simulink model "xor"  (R2015a)
settings: Solver=ode23t  StartTime=0.0  StopTime=1  RelTol=1e-3
libraries: fl_lib x57, nesl_utility x54, elec_lib x5
settings Model: Creator=tomas  LastModifiedBy=tomas

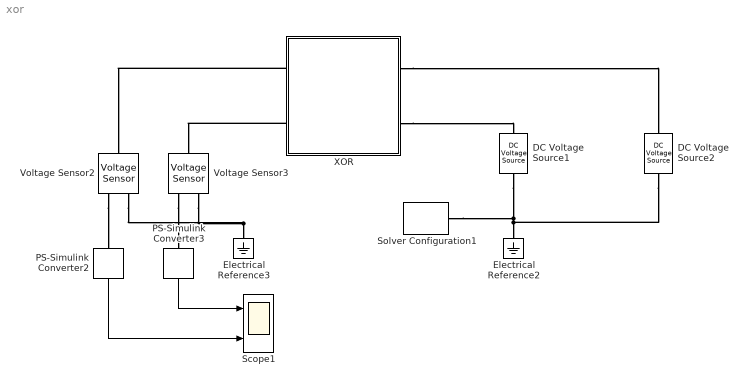
== system xor ==
  DC Voltage Source1 : fl_lib/Electrical/Electrical Sources/DC Voltage Source  v0=1 V
  DC Voltage Source2 : fl_lib/Electrical/Electrical Sources/DC Voltage Source  v0=1 V
  Electrical Reference2 : fl_lib/Electrical/Electrical Elements/Electrical Reference
  Electrical Reference3 : fl_lib/Electrical/Electrical Elements/Electrical Reference
  PS-Simulink Converter2 : nesl_utility/PS-Simulink Converter  PhysicalDomain=network_engine_domain  SubClassName=ps_output  LeftPortType=input  RightPortType=output  PseudoPeriodic=off  Frequencies=[]  Unit=1  AffineConversion=off
  PS-Simulink Converter3 : nesl_utility/PS-Simulink Converter  PhysicalDomain=network_engine_domain  SubClassName=ps_output  LeftPortType=input  RightPortType=output  PseudoPeriodic=off  Frequencies=[]  Unit=1  AffineConversion=off
  Scope1 : Scope  NumInputPorts=2
      settings: YMin=-5~-5  YMax=5~5
  Solver Configuration1 : nesl_utility/Solver Configuration  PhysicalDomain=network_engine_domain  SubClassName=solver  LeftPortType=input  RightPortType=generic  Accelerate=off  Tones=[]  Harmonics=[]  SimulateNoise=off  Profile=off  UseLocalSampling=off  EnableSwitchedLinearOptims=on  FrequencyDomain=off  UseCCode=off  RelTol=0.001  AbsTol=1e-06  MinStep=1e-09  ToWorkspace=off  RevertToSquareIcSolve=off  NumHomotopyIterations=100  DoDC=off  ResidualTolerance=1e-09  UseLocalSolver=off  LocalSolverChoice=NE_BACKWARD_EULER_ADVANCER  LocalSolverSampleTime=0.001  DoFixedCost=off  MaxNonlinIter=3  MaxModeIter=2  LinearAlgebra=Sparse  DelaysMemoryBudget=1024  AutomaticFiltering=on  FilteringTimeConstant=0.001
  Voltage Sensor2 : fl_lib/Electrical/Electrical Sensors/Voltage Sensor
  Voltage Sensor3 : fl_lib/Electrical/Electrical Sensors/Voltage Sensor
  XOR : Subsystem
  wires:
  PS-Simulink Converter3/1 -> Scope1/1
  PS-Simulink Converter2/1 -> Scope1/2
  connections:
  DC Voltage Source1/RConn1 -- Solver Configuration1/RConn1 -- DC Voltage Source2/RConn1 -- Electrical Reference2/LConn1
  Electrical Reference3/LConn1 -- Voltage Sensor3/RConn2 -- Voltage Sensor2/RConn2
  Voltage Sensor2/RConn1 -- PS-Simulink Converter2/LConn1
  XOR/LConn1 -- Voltage Sensor2/LConn1
  XOR/LConn2 -- Voltage Sensor3/LConn1
  Voltage Sensor3/RConn1 -- PS-Simulink Converter3/LConn1
  XOR/RConn2 -- DC Voltage Source1/LConn1
  XOR/RConn1 -- DC Voltage Source2/LConn1

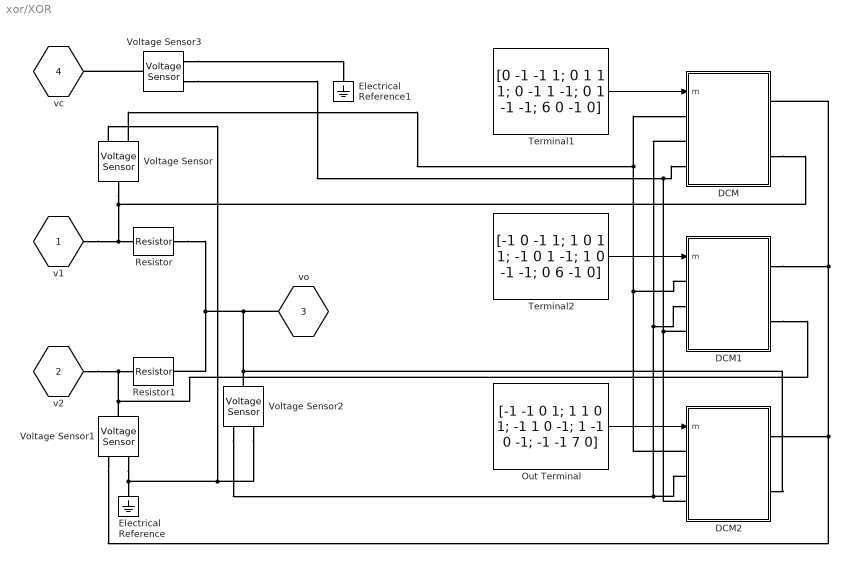
== system xor/XOR ==
  DCM : Subsystem
  DCM1 : Subsystem
  DCM2 : Subsystem
  Electrical Reference : fl_lib/Electrical/Electrical Elements/Electrical Reference
  Electrical Reference1 : fl_lib/Electrical/Electrical Elements/Electrical Reference
  Out Terminal : Constant  Value=[-1 -1 0 1; 1 1 0 1; -1 1 0 -1; 1 -1 0 -1; -1 -1 7 0]  VectorParams1D=off
  Resistor : elec_lib/Passive Devices/Resistor  R=16 kOhm  noise_mode=0  Tdevice=25 C  sample_time=0.001 s  repeatability=1  auto_seed=3002755773  user_seed=0
  Resistor1 : elec_lib/Passive Devices/Resistor  R=16 kOhm  noise_mode=0  Tdevice=25 C  sample_time=0.001 s  repeatability=1  auto_seed=3419901825  user_seed=0
  Terminal1 : Constant  Value=[0 -1 -1 1; 0 1 1 1; 0 -1 1 -1; 0 1 -1 -1; 6 0 -1 0]  VectorParams1D=off
  Terminal2 : Constant  Value=[-1 0 -1 1; 1 0 1 1; -1 0 1 -1; 1 0 -1 -1; 0 6 -1 0]  VectorParams1D=off
  Voltage Sensor{,1..3} (4 alike) : fl_lib/Electrical/Electrical Sensors/Voltage Sensor
  v1 : PMIOPort  Port=1  Side=Left
  v2 : PMIOPort  Port=2  Side=Left
  vo : PMIOPort  Port=3  Side=Right
  vc : PMIOPort  Port=4  Side=Right
  wires:
  Terminal2/1 -> DCM1/1(m)
  Out Terminal/1 -> DCM2/1(m)
  Terminal1/1 -> DCM/1(m)
  connections:
  DCM/RConn2 -- Voltage Sensor/LConn1 -- Resistor/LConn1 -- v1/RConn1
  DCM1/RConn2 -- Voltage Sensor1/LConn1 -- Resistor1/LConn1 -- v2/RConn1
  DCM2/RConn1 -- DCM1/RConn1 -- DCM/RConn1 -- Voltage Sensor1/RConn1
  DCM2/LConn1 -- DCM1/LConn1 -- DCM/LConn1 -- Voltage Sensor/RConn1
  DCM2/RConn2 -- Voltage Sensor2/LConn1 -- Resistor/RConn1 -- Resistor1/RConn1 -- vo/RConn1
  Voltage Sensor2/RConn2 -- Voltage Sensor1/RConn2 -- Electrical Reference/LConn1 -- Voltage Sensor/RConn2
  DCM2/LConn2 -- DCM/LConn2 -- DCM1/LConn2 -- Voltage Sensor2/RConn1
  Voltage Sensor3/LConn1 -- vc/RConn1
  DCM1/LConn3 -- DCM/LConn3 -- Voltage Sensor3/RConn1 -- DCM2/LConn3
  Voltage Sensor3/RConn2 -- Electrical Reference1/LConn1

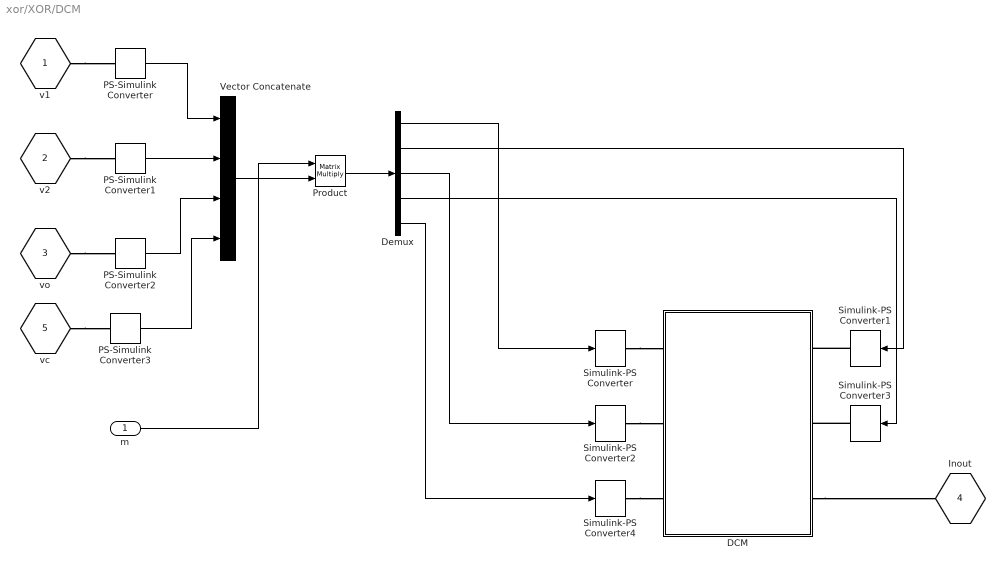
== system xor/XOR/DCM ==
  m : Inport
  DCM : Subsystem
  Demux : Demux  Outputs=5
  PS-Simulink Converter{,1..3} (4 alike) : nesl_utility/PS-Simulink Converter  PhysicalDomain=network_engine_domain  SubClassName=ps_output  LeftPortType=input  RightPortType=output  PseudoPeriodic=off  Frequencies=[]  Unit=V  AffineConversion=off
  Product : Product  Multiplication=Matrix(*)
  Simulink-PS Converter{,1..4} (5 alike) : nesl_utility/Simulink-PS Converter  PhysicalDomain=network_engine_domain  SubClassName=ps_input  LeftPortType=input  RightPortType=output  PseudoPeriodic=off  Frequencies=[]  NoiseDistribution=none  NoiseParameters=[]  Unit=V  AffineConversion=off  InputFiltering=off  SimscapeFilterOrder=1  InputFilterTimeConstant=0.001  UdotUserProvided=1
  Vector Concatenate : Concatenate  NumInputs=4
  "v1 " : PMIOPort  Port=1  Side=Left
  v2 : PMIOPort  Port=2  Side=Right
  vo : PMIOPort  Port=3  Side=Left
  Inout : PMIOPort  Port=4  Side=Right
  vc : PMIOPort  Port=5  Side=Left
  wires:
  Demux/5 -> Simulink-PS Converter4/1
  PS-Simulink Converter3/1 -> Vector Concatenate/4
  Demux/3 -> Simulink-PS Converter2/1
  PS-Simulink Converter/1 -> Vector Concatenate/1
  PS-Simulink Converter2/1 -> Vector Concatenate/3
  PS-Simulink Converter1/1 -> Vector Concatenate/2
  Demux/1 -> Simulink-PS Converter/1
  Demux/4 -> Simulink-PS Converter3/1
  m/1 -> Product/1
  Vector Concatenate/1 -> Product/2
  Product/1 -> Demux/1
  Demux/2 -> Simulink-PS Converter1/1
  connections:
  Simulink-PS Converter2/RConn1 -- DCM/LConn2
  DCM/RConn3 -- Inout/RConn1
  Simulink-PS Converter3/RConn1 -- DCM/RConn2
  vo/RConn1 -- PS-Simulink Converter2/LConn1
  Simulink-PS Converter4/RConn1 -- DCM/LConn3
  Simulink-PS Converter/RConn1 -- DCM/LConn1
  "v1 "/RConn1 -- PS-Simulink Converter/LConn1
  v2/RConn1 -- PS-Simulink Converter1/LConn1
  Simulink-PS Converter1/RConn1 -- DCM/RConn1
  vc/RConn1 -- PS-Simulink Converter3/LConn1

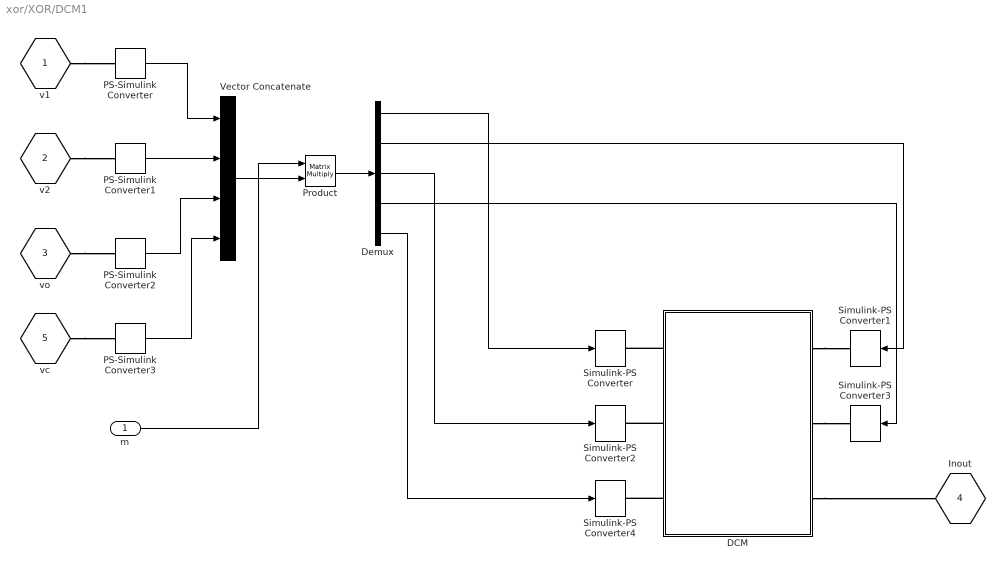
== system xor/XOR/DCM1 ==
  m : Inport
  DCM : Subsystem
  Demux : Demux  Outputs=5
  PS-Simulink Converter{,1..3} (4 alike) : nesl_utility/PS-Simulink Converter  PhysicalDomain=network_engine_domain  SubClassName=ps_output  LeftPortType=input  RightPortType=output  PseudoPeriodic=off  Frequencies=[]  Unit=V  AffineConversion=off
  Product : Product  Multiplication=Matrix(*)
  Simulink-PS Converter{,1..4} (5 alike) : nesl_utility/Simulink-PS Converter  PhysicalDomain=network_engine_domain  SubClassName=ps_input  LeftPortType=input  RightPortType=output  PseudoPeriodic=off  Frequencies=[]  NoiseDistribution=none  NoiseParameters=[]  Unit=V  AffineConversion=off  InputFiltering=off  SimscapeFilterOrder=1  InputFilterTimeConstant=0.001  UdotUserProvided=1
  Vector Concatenate : Concatenate  NumInputs=4
  "v1 " : PMIOPort  Port=1  Side=Left
  v2 : PMIOPort  Port=2  Side=Right
  vo : PMIOPort  Port=3  Side=Left
  Inout : PMIOPort  Port=4  Side=Right
  vc : PMIOPort  Port=5  Side=Left
  wires:
  Demux/5 -> Simulink-PS Converter4/1
  Demux/3 -> Simulink-PS Converter2/1
  PS-Simulink Converter/1 -> Vector Concatenate/1
  PS-Simulink Converter2/1 -> Vector Concatenate/3
  Demux/2 -> Simulink-PS Converter1/1
  PS-Simulink Converter1/1 -> Vector Concatenate/2
  Demux/1 -> Simulink-PS Converter/1
  Demux/4 -> Simulink-PS Converter3/1
  m/1 -> Product/1
  Vector Concatenate/1 -> Product/2
  Product/1 -> Demux/1
  PS-Simulink Converter3/1 -> Vector Concatenate/4
  connections:
  DCM/LConn2 -- Simulink-PS Converter2/RConn1
  vo/RConn1 -- PS-Simulink Converter2/LConn1
  DCM/LConn3 -- Simulink-PS Converter4/RConn1
  DCM/LConn1 -- Simulink-PS Converter/RConn1
  "v1 "/RConn1 -- PS-Simulink Converter/LConn1
  v2/RConn1 -- PS-Simulink Converter1/LConn1
  vc/RConn1 -- PS-Simulink Converter3/LConn1
  DCM/RConn1 -- Simulink-PS Converter1/RConn1
  DCM/RConn2 -- Simulink-PS Converter3/RConn1
  DCM/RConn3 -- Inout/RConn1

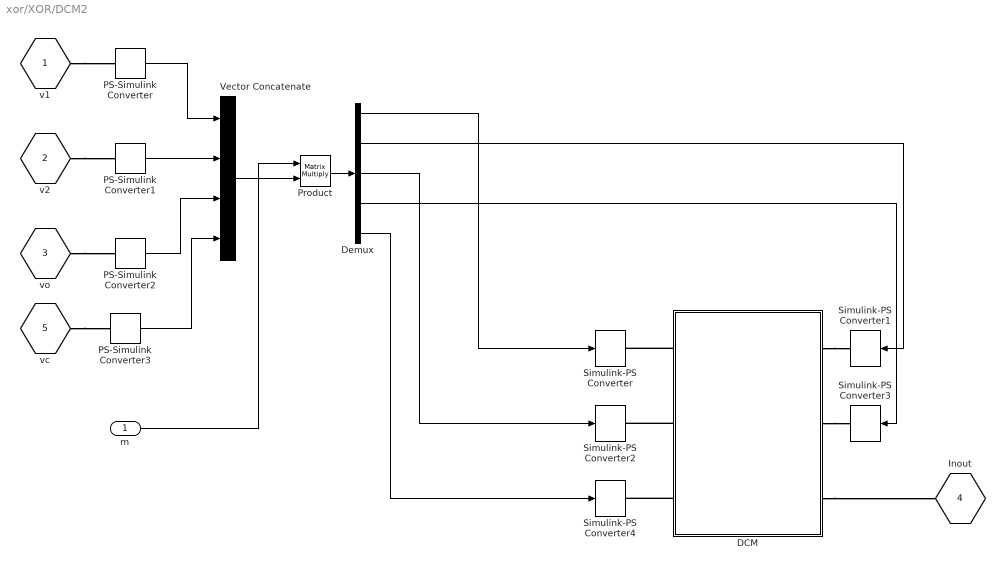
== system xor/XOR/DCM2 ==
  m : Inport
  DCM : Subsystem
  Demux : Demux  Outputs=5
  PS-Simulink Converter{,1..3} (4 alike) : nesl_utility/PS-Simulink Converter  PhysicalDomain=network_engine_domain  SubClassName=ps_output  LeftPortType=input  RightPortType=output  PseudoPeriodic=off  Frequencies=[]  Unit=V  AffineConversion=off
  Product : Product  Multiplication=Matrix(*)
  Simulink-PS Converter{,1..4} (5 alike) : nesl_utility/Simulink-PS Converter  PhysicalDomain=network_engine_domain  SubClassName=ps_input  LeftPortType=input  RightPortType=output  PseudoPeriodic=off  Frequencies=[]  NoiseDistribution=none  NoiseParameters=[]  Unit=V  AffineConversion=off  InputFiltering=off  SimscapeFilterOrder=1  InputFilterTimeConstant=0.001  UdotUserProvided=1
  Vector Concatenate : Concatenate  NumInputs=4
  "v1 " : PMIOPort  Port=1  Side=Left
  v2 : PMIOPort  Port=2  Side=Right
  vo : PMIOPort  Port=3  Side=Left
  Inout : PMIOPort  Port=4  Side=Right
  vc : PMIOPort  Port=5  Side=Left
  wires:
  Demux/5 -> Simulink-PS Converter4/1
  Demux/3 -> Simulink-PS Converter2/1
  PS-Simulink Converter/1 -> Vector Concatenate/1
  PS-Simulink Converter2/1 -> Vector Concatenate/3
  Demux/2 -> Simulink-PS Converter1/1
  PS-Simulink Converter1/1 -> Vector Concatenate/2
  Demux/1 -> Simulink-PS Converter/1
  Demux/4 -> Simulink-PS Converter3/1
  m/1 -> Product/1
  Vector Concatenate/1 -> Product/2
  Product/1 -> Demux/1
  PS-Simulink Converter3/1 -> Vector Concatenate/4
  connections:
  DCM/LConn2 -- Simulink-PS Converter2/RConn1
  vo/RConn1 -- PS-Simulink Converter2/LConn1
  DCM/LConn3 -- Simulink-PS Converter4/RConn1
  DCM/LConn1 -- Simulink-PS Converter/RConn1
  "v1 "/RConn1 -- PS-Simulink Converter/LConn1
  v2/RConn1 -- PS-Simulink Converter1/LConn1
  vc/RConn1 -- PS-Simulink Converter3/LConn1
  DCM/RConn1 -- Simulink-PS Converter1/RConn1
  DCM/RConn2 -- Simulink-PS Converter3/RConn1
  DCM/RConn3 -- Inout/RConn1

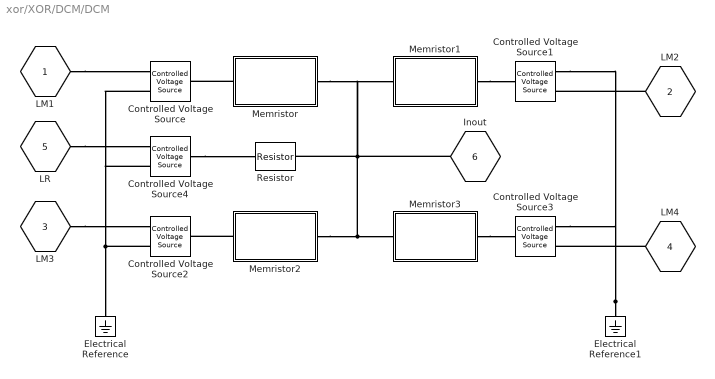
== system xor/XOR/DCM/DCM ==
  Controlled Voltage Source{,1..4} (5 alike) : fl_lib/Electrical/Electrical Sources/Controlled Voltage Source
  Electrical Reference : fl_lib/Electrical/Electrical Elements/Electrical Reference
  Electrical Reference1 : fl_lib/Electrical/Electrical Elements/Electrical Reference
  Memristor : Subsystem  Tag=Memristor
  Memristor1 : Subsystem  Tag=Memristor
  Memristor2 : Subsystem  Tag=Memristor
  Memristor3 : Subsystem  Tag=Memristor
  Resistor : elec_lib/Passive Devices/Resistor  R=16 kOhm  noise_mode=0  Tdevice=25 C  sample_time=0.001 s  repeatability=1  auto_seed=2451064179  user_seed=0
  LM1 : PMIOPort  Port=1  Side=Left
  LM2 : PMIOPort  Port=2  Side=Right
  LM3 : PMIOPort  Port=3  Side=Left
  LM4 : PMIOPort  Port=4  Side=Right
  LR : PMIOPort  Port=5  Side=Left
  Inout : PMIOPort  Port=6  Side=Right
  connections:
  LM2/RConn1 -- Controlled Voltage Source1/RConn1
  Controlled Voltage Source2/RConn2 -- Electrical Reference/LConn1 -- Controlled Voltage Source/RConn2 -- Controlled Voltage Source4/RConn2
  Controlled Voltage Source4/LConn1 -- Resistor/LConn1
  Memristor2/RConn1 -- Memristor1/LConn1 -- Memristor/LConn1 -- Resistor/RConn1 -- Inout/RConn1 -- Memristor3/RConn1
  Electrical Reference1/LConn1 -- Controlled Voltage Source1/RConn2 -- Controlled Voltage Source3/RConn2
  LM1/RConn1 -- Controlled Voltage Source/RConn1
  LM4/RConn1 -- Controlled Voltage Source3/RConn1
  LR/RConn1 -- Controlled Voltage Source4/RConn1
  LM3/RConn1 -- Controlled Voltage Source2/RConn1
  Memristor2/LConn1 -- Controlled Voltage Source2/LConn1
  Memristor3/LConn1 -- Controlled Voltage Source3/LConn1
  Memristor1/RConn1 -- Controlled Voltage Source1/LConn1
  Memristor/RConn1 -- Controlled Voltage Source/LConn1

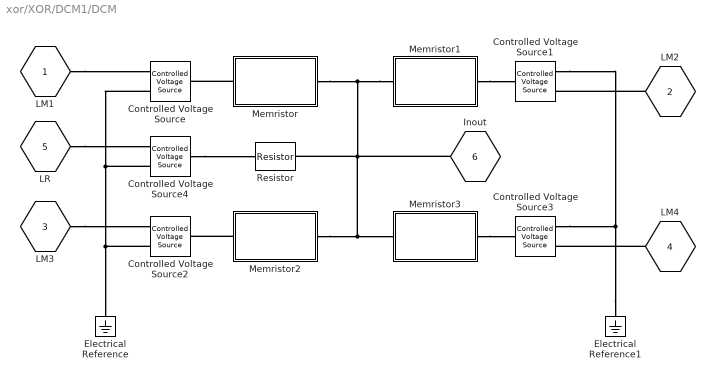
== system xor/XOR/DCM1/DCM ==
  Controlled Voltage Source{,1..4} (5 alike) : fl_lib/Electrical/Electrical Sources/Controlled Voltage Source
  Electrical Reference : fl_lib/Electrical/Electrical Elements/Electrical Reference
  Electrical Reference1 : fl_lib/Electrical/Electrical Elements/Electrical Reference
  Memristor : Subsystem  Tag=Memristor
  Memristor1 : Subsystem  Tag=Memristor
  Memristor2 : Subsystem  Tag=Memristor
  Memristor3 : Subsystem  Tag=Memristor
  Resistor : elec_lib/Passive Devices/Resistor  R=16 kOhm  noise_mode=0  Tdevice=25 C  sample_time=0.001 s  repeatability=1  auto_seed=1880221209  user_seed=0
  LM1 : PMIOPort  Port=1  Side=Left
  LM2 : PMIOPort  Port=2  Side=Right
  LM3 : PMIOPort  Port=3  Side=Left
  LM4 : PMIOPort  Port=4  Side=Right
  LR : PMIOPort  Port=5  Side=Left
  Inout : PMIOPort  Port=6  Side=Right
  connections:
  LM2/RConn1 -- Controlled Voltage Source1/RConn1
  Controlled Voltage Source2/RConn2 -- Electrical Reference/LConn1 -- Controlled Voltage Source/RConn2 -- Controlled Voltage Source4/RConn2
  Controlled Voltage Source4/LConn1 -- Resistor/LConn1
  Memristor1/LConn1 -- Memristor/LConn1 -- Resistor/RConn1 -- Inout/RConn1 -- Memristor2/RConn1 -- Memristor3/RConn1
  Electrical Reference1/LConn1 -- Controlled Voltage Source1/RConn2 -- Controlled Voltage Source3/RConn2
  LM1/RConn1 -- Controlled Voltage Source/RConn1
  LM4/RConn1 -- Controlled Voltage Source3/RConn1
  LR/RConn1 -- Controlled Voltage Source4/RConn1
  LM3/RConn1 -- Controlled Voltage Source2/RConn1
  Memristor2/LConn1 -- Controlled Voltage Source2/LConn1
  Memristor3/LConn1 -- Controlled Voltage Source3/LConn1
  Memristor1/RConn1 -- Controlled Voltage Source1/LConn1
  Memristor/RConn1 -- Controlled Voltage Source/LConn1

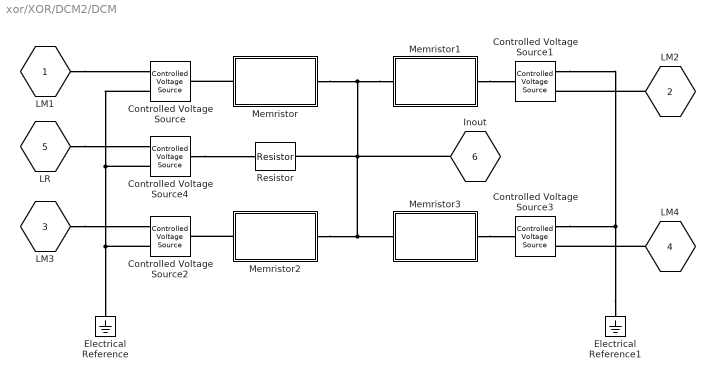
== system xor/XOR/DCM2/DCM ==
  Controlled Voltage Source{,1..4} (5 alike) : fl_lib/Electrical/Electrical Sources/Controlled Voltage Source
  Electrical Reference : fl_lib/Electrical/Electrical Elements/Electrical Reference
  Electrical Reference1 : fl_lib/Electrical/Electrical Elements/Electrical Reference
  Memristor : Subsystem  Tag=Memristor
  Memristor1 : Subsystem  Tag=Memristor
  Memristor2 : Subsystem  Tag=Memristor
  Memristor3 : Subsystem  Tag=Memristor
  Resistor : elec_lib/Passive Devices/Resistor  R=16 kOhm  noise_mode=0  Tdevice=25 C  sample_time=0.001 s  repeatability=1  auto_seed=1203579070  user_seed=0
  LM1 : PMIOPort  Port=1  Side=Left
  LM2 : PMIOPort  Port=2  Side=Right
  LM3 : PMIOPort  Port=3  Side=Left
  LM4 : PMIOPort  Port=4  Side=Right
  LR : PMIOPort  Port=5  Side=Left
  Inout : PMIOPort  Port=6  Side=Right
  connections:
  LM2/RConn1 -- Controlled Voltage Source1/RConn1
  Controlled Voltage Source2/RConn2 -- Electrical Reference/LConn1 -- Controlled Voltage Source/RConn2 -- Controlled Voltage Source4/RConn2
  Controlled Voltage Source4/LConn1 -- Resistor/LConn1
  Memristor1/LConn1 -- Memristor/LConn1 -- Resistor/RConn1 -- Inout/RConn1 -- Memristor2/RConn1 -- Memristor3/RConn1
  Electrical Reference1/LConn1 -- Controlled Voltage Source1/RConn2 -- Controlled Voltage Source3/RConn2
  LM1/RConn1 -- Controlled Voltage Source/RConn1
  LM4/RConn1 -- Controlled Voltage Source3/RConn1
  LR/RConn1 -- Controlled Voltage Source4/RConn1
  LM3/RConn1 -- Controlled Voltage Source2/RConn1
  Memristor2/LConn1 -- Controlled Voltage Source2/LConn1
  Memristor3/LConn1 -- Controlled Voltage Source3/LConn1
  Memristor1/RConn1 -- Controlled Voltage Source1/LConn1
  Memristor/RConn1 -- Controlled Voltage Source/LConn1

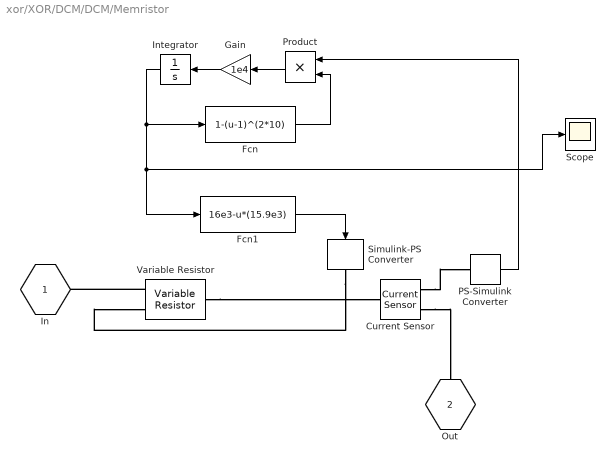
== system xor/XOR/DCM/DCM/Memristor ==
  Current Sensor : fl_lib/Electrical/Electrical Sensors/Current Sensor
  Fcn : Fcn  Expr=1-(u-1)^(2*10)
  Fcn1 : Fcn  Expr=16e3-u*(15.9e3)
  Gain : Gain  Gain=1e4
  Integrator : Integrator  InitialCondition=rand()
  PS-Simulink Converter : nesl_utility/PS-Simulink Converter  PhysicalDomain=network_engine_domain  SubClassName=ps_output  LeftPortType=input  RightPortType=output  PseudoPeriodic=off  Frequencies=[]  Unit=1  AffineConversion=off
  Product : Product
  Scope : Scope
  Simulink-PS Converter : nesl_utility/Simulink-PS Converter  PhysicalDomain=network_engine_domain  SubClassName=ps_input  LeftPortType=input  RightPortType=output  PseudoPeriodic=off  Frequencies=[]  NoiseDistribution=none  NoiseParameters=[]  Unit=1  AffineConversion=off  InputFiltering=off  SimscapeFilterOrder=1  InputFilterTimeConstant=0.001  UdotUserProvided=1
  Variable Resistor : fl_lib/Electrical/Electrical Elements/Variable Resistor  Rmin=100 Ohm  i_specify=off  i_priority=High  i=0 A  v_specify=off  v_priority=High  v=0 V
  In : PMIOPort  Port=1  Side=Left
  Out : PMIOPort  Port=2  Side=Right
  wires:
  Gain/1 -> Integrator/1
  Product/1 -> Gain/1
  Integrator/1 -> Scope/1, Fcn1/1, Fcn/1
  Fcn/1 -> Product/2
  Fcn1/1 -> Simulink-PS Converter/1
  PS-Simulink Converter/1 -> Product/1
  connections:
  Current Sensor/RConn1 -- PS-Simulink Converter/LConn1
  Simulink-PS Converter/RConn1 -- Variable Resistor/LConn1
  Current Sensor/RConn2 -- Out/RConn1
  Variable Resistor/RConn1 -- Current Sensor/LConn1
  Variable Resistor/LConn2 -- In/RConn1

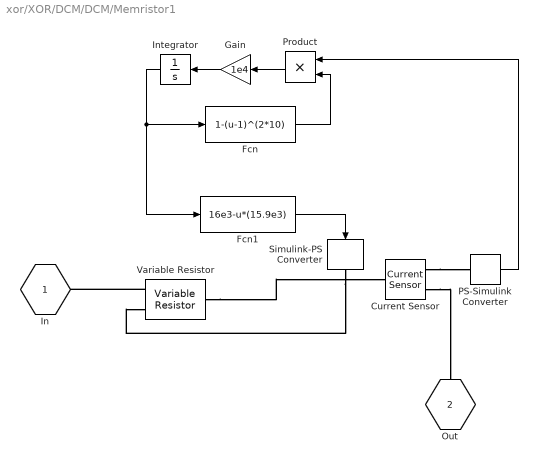
== system xor/XOR/DCM/DCM/Memristor1 ==
  Current Sensor : fl_lib/Electrical/Electrical Sensors/Current Sensor
  Fcn : Fcn  Expr=1-(u-1)^(2*10)
  Fcn1 : Fcn  Expr=16e3-u*(15.9e3)
  Gain : Gain  Gain=1e4
  Integrator : Integrator  InitialCondition=rand()
  PS-Simulink Converter : nesl_utility/PS-Simulink Converter  PhysicalDomain=network_engine_domain  SubClassName=ps_output  LeftPortType=input  RightPortType=output  PseudoPeriodic=off  Frequencies=[]  Unit=1  AffineConversion=off
  Product : Product
  Simulink-PS Converter : nesl_utility/Simulink-PS Converter  PhysicalDomain=network_engine_domain  SubClassName=ps_input  LeftPortType=input  RightPortType=output  PseudoPeriodic=off  Frequencies=[]  NoiseDistribution=none  NoiseParameters=[]  Unit=1  AffineConversion=off  InputFiltering=off  SimscapeFilterOrder=1  InputFilterTimeConstant=0.001  UdotUserProvided=1
  Variable Resistor : fl_lib/Electrical/Electrical Elements/Variable Resistor  Rmin=100 Ohm  i_specify=off  i_priority=High  i=0 A  v_specify=off  v_priority=High  v=0 V
  In : PMIOPort  Port=1  Side=Left
  Out : PMIOPort  Port=2  Side=Right
  wires:
  Gain/1 -> Integrator/1
  Product/1 -> Gain/1
  Integrator/1 -> Fcn1/1, Fcn/1
  Fcn/1 -> Product/2
  Fcn1/1 -> Simulink-PS Converter/1
  PS-Simulink Converter/1 -> Product/1
  connections:
  Variable Resistor/LConn2 -- In/RConn1
  Current Sensor/RConn1 -- PS-Simulink Converter/LConn1
  Current Sensor/RConn2 -- Out/RConn1
  Simulink-PS Converter/RConn1 -- Variable Resistor/LConn1
  Variable Resistor/RConn1 -- Current Sensor/LConn1

== system xor/XOR/DCM/DCM/Memristor2 ==
  Current Sensor : fl_lib/Electrical/Electrical Sensors/Current Sensor
  Fcn : Fcn  Expr=1-(u-1)^(2*10)
  Fcn1 : Fcn  Expr=16e3-u*(15.9e3)
  Gain : Gain  Gain=1e4
  Integrator : Integrator  InitialCondition=rand()
  PS-Simulink Converter : nesl_utility/PS-Simulink Converter  PhysicalDomain=network_engine_domain  SubClassName=ps_output  LeftPortType=input  RightPortType=output  PseudoPeriodic=off  Frequencies=[]  Unit=1  AffineConversion=off
  Product : Product
  Simulink-PS Converter : nesl_utility/Simulink-PS Converter  PhysicalDomain=network_engine_domain  SubClassName=ps_input  LeftPortType=input  RightPortType=output  PseudoPeriodic=off  Frequencies=[]  NoiseDistribution=none  NoiseParameters=[]  Unit=1  AffineConversion=off  InputFiltering=off  SimscapeFilterOrder=1  InputFilterTimeConstant=0.001  UdotUserProvided=1
  Variable Resistor : fl_lib/Electrical/Electrical Elements/Variable Resistor  Rmin=100 Ohm  i_specify=off  i_priority=High  i=0 A  v_specify=off  v_priority=High  v=0 V
  In : PMIOPort  Port=1  Side=Left
  Out : PMIOPort  Port=2  Side=Right
  wires:
  Gain/1 -> Integrator/1
  Product/1 -> Gain/1
  Integrator/1 -> Fcn1/1, Fcn/1
  Fcn/1 -> Product/2
  Fcn1/1 -> Simulink-PS Converter/1
  PS-Simulink Converter/1 -> Product/1
  connections:
  Variable Resistor/LConn2 -- In/RConn1
  Current Sensor/RConn1 -- PS-Simulink Converter/LConn1
  Current Sensor/RConn2 -- Out/RConn1
  Variable Resistor/RConn1 -- Current Sensor/LConn1
  Simulink-PS Converter/RConn1 -- Variable Resistor/LConn1

== system xor/XOR/DCM/DCM/Memristor3 ==
  Current Sensor : fl_lib/Electrical/Electrical Sensors/Current Sensor
  Fcn : Fcn  Expr=1-(u-1)^(2*10)
  Fcn1 : Fcn  Expr=16e3-u*(15.9e3)
  Gain : Gain  Gain=1e4
  Integrator : Integrator  InitialCondition=rand()
  PS-Simulink Converter : nesl_utility/PS-Simulink Converter  PhysicalDomain=network_engine_domain  SubClassName=ps_output  LeftPortType=input  RightPortType=output  PseudoPeriodic=off  Frequencies=[]  Unit=1  AffineConversion=off
  Product : Product
  Simulink-PS Converter : nesl_utility/Simulink-PS Converter  PhysicalDomain=network_engine_domain  SubClassName=ps_input  LeftPortType=input  RightPortType=output  PseudoPeriodic=off  Frequencies=[]  NoiseDistribution=none  NoiseParameters=[]  Unit=1  AffineConversion=off  InputFiltering=off  SimscapeFilterOrder=1  InputFilterTimeConstant=0.001  UdotUserProvided=1
  Variable Resistor : fl_lib/Electrical/Electrical Elements/Variable Resistor  Rmin=100 Ohm  i_specify=off  i_priority=High  i=0 A  v_specify=off  v_priority=High  v=0 V
  In : PMIOPort  Port=1  Side=Left
  Out : PMIOPort  Port=2  Side=Right
  wires:
  Gain/1 -> Integrator/1
  Product/1 -> Gain/1
  Integrator/1 -> Fcn1/1, Fcn/1
  Fcn/1 -> Product/2
  Fcn1/1 -> Simulink-PS Converter/1
  PS-Simulink Converter/1 -> Product/1
  connections:
  Current Sensor/RConn1 -- PS-Simulink Converter/LConn1
  Current Sensor/RConn2 -- Out/RConn1
  Variable Resistor/LConn2 -- In/RConn1
  Simulink-PS Converter/RConn1 -- Variable Resistor/LConn1
  Variable Resistor/RConn1 -- Current Sensor/LConn1

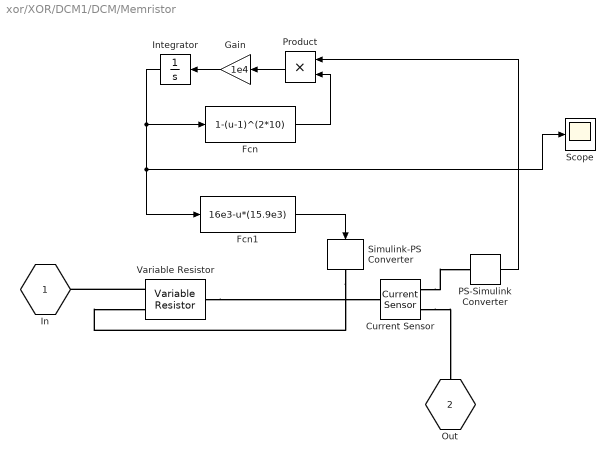
== system xor/XOR/DCM1/DCM/Memristor ==
  Current Sensor : fl_lib/Electrical/Electrical Sensors/Current Sensor
  Fcn : Fcn  Expr=1-(u-1)^(2*10)
  Fcn1 : Fcn  Expr=16e3-u*(15.9e3)
  Gain : Gain  Gain=1e4
  Integrator : Integrator  InitialCondition=rand()
  PS-Simulink Converter : nesl_utility/PS-Simulink Converter  PhysicalDomain=network_engine_domain  SubClassName=ps_output  LeftPortType=input  RightPortType=output  PseudoPeriodic=off  Frequencies=[]  Unit=1  AffineConversion=off
  Product : Product
  Scope : Scope
  Simulink-PS Converter : nesl_utility/Simulink-PS Converter  PhysicalDomain=network_engine_domain  SubClassName=ps_input  LeftPortType=input  RightPortType=output  PseudoPeriodic=off  Frequencies=[]  NoiseDistribution=none  NoiseParameters=[]  Unit=1  AffineConversion=off  InputFiltering=off  SimscapeFilterOrder=1  InputFilterTimeConstant=0.001  UdotUserProvided=1
  Variable Resistor : fl_lib/Electrical/Electrical Elements/Variable Resistor  Rmin=100 Ohm  i_specify=off  i_priority=High  i=0 A  v_specify=off  v_priority=High  v=0 V
  In : PMIOPort  Port=1  Side=Left
  Out : PMIOPort  Port=2  Side=Right
  wires:
  Gain/1 -> Integrator/1
  Product/1 -> Gain/1
  Integrator/1 -> Scope/1, Fcn1/1, Fcn/1
  Fcn/1 -> Product/2
  Fcn1/1 -> Simulink-PS Converter/1
  PS-Simulink Converter/1 -> Product/1
  connections:
  Current Sensor/RConn1 -- PS-Simulink Converter/LConn1
  Simulink-PS Converter/RConn1 -- Variable Resistor/LConn1
  Current Sensor/RConn2 -- Out/RConn1
  Variable Resistor/RConn1 -- Current Sensor/LConn1
  Variable Resistor/LConn2 -- In/RConn1

== system xor/XOR/DCM1/DCM/Memristor1 ==
  Current Sensor : fl_lib/Electrical/Electrical Sensors/Current Sensor
  Fcn : Fcn  Expr=1-(u-1)^(2*10)
  Fcn1 : Fcn  Expr=16e3-u*(15.9e3)
  Gain : Gain  Gain=1e4
  Integrator : Integrator  InitialCondition=rand()
  PS-Simulink Converter : nesl_utility/PS-Simulink Converter  PhysicalDomain=network_engine_domain  SubClassName=ps_output  LeftPortType=input  RightPortType=output  PseudoPeriodic=off  Frequencies=[]  Unit=1  AffineConversion=off
  Product : Product
  Simulink-PS Converter : nesl_utility/Simulink-PS Converter  PhysicalDomain=network_engine_domain  SubClassName=ps_input  LeftPortType=input  RightPortType=output  PseudoPeriodic=off  Frequencies=[]  NoiseDistribution=none  NoiseParameters=[]  Unit=1  AffineConversion=off  InputFiltering=off  SimscapeFilterOrder=1  InputFilterTimeConstant=0.001  UdotUserProvided=1
  Variable Resistor : fl_lib/Electrical/Electrical Elements/Variable Resistor  Rmin=100 Ohm  i_specify=off  i_priority=High  i=0 A  v_specify=off  v_priority=High  v=0 V
  In : PMIOPort  Port=1  Side=Left
  Out : PMIOPort  Port=2  Side=Right
  wires:
  Gain/1 -> Integrator/1
  Product/1 -> Gain/1
  Integrator/1 -> Fcn1/1, Fcn/1
  Fcn/1 -> Product/2
  Fcn1/1 -> Simulink-PS Converter/1
  PS-Simulink Converter/1 -> Product/1
  connections:
  Variable Resistor/LConn2 -- In/RConn1
  Current Sensor/RConn1 -- PS-Simulink Converter/LConn1
  Current Sensor/RConn2 -- Out/RConn1
  Simulink-PS Converter/RConn1 -- Variable Resistor/LConn1
  Variable Resistor/RConn1 -- Current Sensor/LConn1

== system xor/XOR/DCM1/DCM/Memristor2 ==
  Current Sensor : fl_lib/Electrical/Electrical Sensors/Current Sensor
  Fcn : Fcn  Expr=1-(u-1)^(2*10)
  Fcn1 : Fcn  Expr=16e3-u*(15.9e3)
  Gain : Gain  Gain=1e4
  Integrator : Integrator  InitialCondition=rand()
  PS-Simulink Converter : nesl_utility/PS-Simulink Converter  PhysicalDomain=network_engine_domain  SubClassName=ps_output  LeftPortType=input  RightPortType=output  PseudoPeriodic=off  Frequencies=[]  Unit=1  AffineConversion=off
  Product : Product
  Simulink-PS Converter : nesl_utility/Simulink-PS Converter  PhysicalDomain=network_engine_domain  SubClassName=ps_input  LeftPortType=input  RightPortType=output  PseudoPeriodic=off  Frequencies=[]  NoiseDistribution=none  NoiseParameters=[]  Unit=1  AffineConversion=off  InputFiltering=off  SimscapeFilterOrder=1  InputFilterTimeConstant=0.001  UdotUserProvided=1
  Variable Resistor : fl_lib/Electrical/Electrical Elements/Variable Resistor  Rmin=100 Ohm  i_specify=off  i_priority=High  i=0 A  v_specify=off  v_priority=High  v=0 V
  In : PMIOPort  Port=1  Side=Left
  Out : PMIOPort  Port=2  Side=Right
  wires:
  Gain/1 -> Integrator/1
  Product/1 -> Gain/1
  Integrator/1 -> Fcn1/1, Fcn/1
  Fcn/1 -> Product/2
  Fcn1/1 -> Simulink-PS Converter/1
  PS-Simulink Converter/1 -> Product/1
  connections:
  Variable Resistor/LConn2 -- In/RConn1
  Current Sensor/RConn1 -- PS-Simulink Converter/LConn1
  Current Sensor/RConn2 -- Out/RConn1
  Variable Resistor/RConn1 -- Current Sensor/LConn1
  Simulink-PS Converter/RConn1 -- Variable Resistor/LConn1

== system xor/XOR/DCM1/DCM/Memristor3 ==
  Current Sensor : fl_lib/Electrical/Electrical Sensors/Current Sensor
  Fcn : Fcn  Expr=1-(u-1)^(2*10)
  Fcn1 : Fcn  Expr=16e3-u*(15.9e3)
  Gain : Gain  Gain=1e4
  Integrator : Integrator  InitialCondition=rand()
  PS-Simulink Converter : nesl_utility/PS-Simulink Converter  PhysicalDomain=network_engine_domain  SubClassName=ps_output  LeftPortType=input  RightPortType=output  PseudoPeriodic=off  Frequencies=[]  Unit=1  AffineConversion=off
  Product : Product
  Simulink-PS Converter : nesl_utility/Simulink-PS Converter  PhysicalDomain=network_engine_domain  SubClassName=ps_input  LeftPortType=input  RightPortType=output  PseudoPeriodic=off  Frequencies=[]  NoiseDistribution=none  NoiseParameters=[]  Unit=1  AffineConversion=off  InputFiltering=off  SimscapeFilterOrder=1  InputFilterTimeConstant=0.001  UdotUserProvided=1
  Variable Resistor : fl_lib/Electrical/Electrical Elements/Variable Resistor  Rmin=100 Ohm  i_specify=off  i_priority=High  i=0 A  v_specify=off  v_priority=High  v=0 V
  In : PMIOPort  Port=1  Side=Left
  Out : PMIOPort  Port=2  Side=Right
  wires:
  Gain/1 -> Integrator/1
  Product/1 -> Gain/1
  Integrator/1 -> Fcn1/1, Fcn/1
  Fcn/1 -> Product/2
  Fcn1/1 -> Simulink-PS Converter/1
  PS-Simulink Converter/1 -> Product/1
  connections:
  Current Sensor/RConn1 -- PS-Simulink Converter/LConn1
  Current Sensor/RConn2 -- Out/RConn1
  Variable Resistor/LConn2 -- In/RConn1
  Simulink-PS Converter/RConn1 -- Variable Resistor/LConn1
  Variable Resistor/RConn1 -- Current Sensor/LConn1

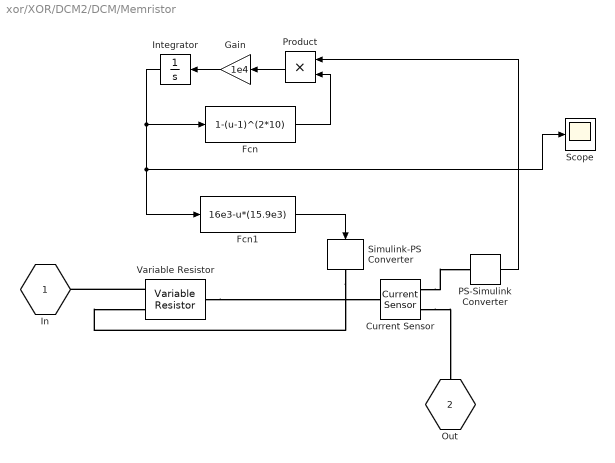
== system xor/XOR/DCM2/DCM/Memristor ==
  Current Sensor : fl_lib/Electrical/Electrical Sensors/Current Sensor
  Fcn : Fcn  Expr=1-(u-1)^(2*10)
  Fcn1 : Fcn  Expr=16e3-u*(15.9e3)
  Gain : Gain  Gain=1e4
  Integrator : Integrator  InitialCondition=rand()
  PS-Simulink Converter : nesl_utility/PS-Simulink Converter  PhysicalDomain=network_engine_domain  SubClassName=ps_output  LeftPortType=input  RightPortType=output  PseudoPeriodic=off  Frequencies=[]  Unit=1  AffineConversion=off
  Product : Product
  Scope : Scope
  Simulink-PS Converter : nesl_utility/Simulink-PS Converter  PhysicalDomain=network_engine_domain  SubClassName=ps_input  LeftPortType=input  RightPortType=output  PseudoPeriodic=off  Frequencies=[]  NoiseDistribution=none  NoiseParameters=[]  Unit=1  AffineConversion=off  InputFiltering=off  SimscapeFilterOrder=1  InputFilterTimeConstant=0.001  UdotUserProvided=1
  Variable Resistor : fl_lib/Electrical/Electrical Elements/Variable Resistor  Rmin=100 Ohm  i_specify=off  i_priority=High  i=0 A  v_specify=off  v_priority=High  v=0 V
  In : PMIOPort  Port=1  Side=Left
  Out : PMIOPort  Port=2  Side=Right
  wires:
  Gain/1 -> Integrator/1
  Product/1 -> Gain/1
  Integrator/1 -> Scope/1, Fcn1/1, Fcn/1
  Fcn/1 -> Product/2
  Fcn1/1 -> Simulink-PS Converter/1
  PS-Simulink Converter/1 -> Product/1
  connections:
  Current Sensor/RConn1 -- PS-Simulink Converter/LConn1
  Simulink-PS Converter/RConn1 -- Variable Resistor/LConn1
  Current Sensor/RConn2 -- Out/RConn1
  Variable Resistor/RConn1 -- Current Sensor/LConn1
  Variable Resistor/LConn2 -- In/RConn1

== system xor/XOR/DCM2/DCM/Memristor1 ==
  Current Sensor : fl_lib/Electrical/Electrical Sensors/Current Sensor
  Fcn : Fcn  Expr=1-(u-1)^(2*10)
  Fcn1 : Fcn  Expr=16e3-u*(15.9e3)
  Gain : Gain  Gain=1e4
  Integrator : Integrator  InitialCondition=rand()
  PS-Simulink Converter : nesl_utility/PS-Simulink Converter  PhysicalDomain=network_engine_domain  SubClassName=ps_output  LeftPortType=input  RightPortType=output  PseudoPeriodic=off  Frequencies=[]  Unit=1  AffineConversion=off
  Product : Product
  Simulink-PS Converter : nesl_utility/Simulink-PS Converter  PhysicalDomain=network_engine_domain  SubClassName=ps_input  LeftPortType=input  RightPortType=output  PseudoPeriodic=off  Frequencies=[]  NoiseDistribution=none  NoiseParameters=[]  Unit=1  AffineConversion=off  InputFiltering=off  SimscapeFilterOrder=1  InputFilterTimeConstant=0.001  UdotUserProvided=1
  Variable Resistor : fl_lib/Electrical/Electrical Elements/Variable Resistor  Rmin=100 Ohm  i_specify=off  i_priority=High  i=0 A  v_specify=off  v_priority=High  v=0 V
  In : PMIOPort  Port=1  Side=Left
  Out : PMIOPort  Port=2  Side=Right
  wires:
  Gain/1 -> Integrator/1
  Product/1 -> Gain/1
  Integrator/1 -> Fcn1/1, Fcn/1
  Fcn/1 -> Product/2
  Fcn1/1 -> Simulink-PS Converter/1
  PS-Simulink Converter/1 -> Product/1
  connections:
  Variable Resistor/LConn2 -- In/RConn1
  Current Sensor/RConn1 -- PS-Simulink Converter/LConn1
  Current Sensor/RConn2 -- Out/RConn1
  Simulink-PS Converter/RConn1 -- Variable Resistor/LConn1
  Variable Resistor/RConn1 -- Current Sensor/LConn1

== system xor/XOR/DCM2/DCM/Memristor2 ==
  Current Sensor : fl_lib/Electrical/Electrical Sensors/Current Sensor
  Fcn : Fcn  Expr=1-(u-1)^(2*10)
  Fcn1 : Fcn  Expr=16e3-u*(15.9e3)
  Gain : Gain  Gain=1e4
  Integrator : Integrator  InitialCondition=rand()
  PS-Simulink Converter : nesl_utility/PS-Simulink Converter  PhysicalDomain=network_engine_domain  SubClassName=ps_output  LeftPortType=input  RightPortType=output  PseudoPeriodic=off  Frequencies=[]  Unit=1  AffineConversion=off
  Product : Product
  Simulink-PS Converter : nesl_utility/Simulink-PS Converter  PhysicalDomain=network_engine_domain  SubClassName=ps_input  LeftPortType=input  RightPortType=output  PseudoPeriodic=off  Frequencies=[]  NoiseDistribution=none  NoiseParameters=[]  Unit=1  AffineConversion=off  InputFiltering=off  SimscapeFilterOrder=1  InputFilterTimeConstant=0.001  UdotUserProvided=1
  Variable Resistor : fl_lib/Electrical/Electrical Elements/Variable Resistor  Rmin=100 Ohm  i_specify=off  i_priority=High  i=0 A  v_specify=off  v_priority=High  v=0 V
  In : PMIOPort  Port=1  Side=Left
  Out : PMIOPort  Port=2  Side=Right
  wires:
  Gain/1 -> Integrator/1
  Product/1 -> Gain/1
  Integrator/1 -> Fcn1/1, Fcn/1
  Fcn/1 -> Product/2
  Fcn1/1 -> Simulink-PS Converter/1
  PS-Simulink Converter/1 -> Product/1
  connections:
  Variable Resistor/LConn2 -- In/RConn1
  Current Sensor/RConn1 -- PS-Simulink Converter/LConn1
  Current Sensor/RConn2 -- Out/RConn1
  Variable Resistor/RConn1 -- Current Sensor/LConn1
  Simulink-PS Converter/RConn1 -- Variable Resistor/LConn1

== system xor/XOR/DCM2/DCM/Memristor3 ==
  Current Sensor : fl_lib/Electrical/Electrical Sensors/Current Sensor
  Fcn : Fcn  Expr=1-(u-1)^(2*10)
  Fcn1 : Fcn  Expr=16e3-u*(15.9e3)
  Gain : Gain  Gain=1e4
  Integrator : Integrator  InitialCondition=rand()
  PS-Simulink Converter : nesl_utility/PS-Simulink Converter  PhysicalDomain=network_engine_domain  SubClassName=ps_output  LeftPortType=input  RightPortType=output  PseudoPeriodic=off  Frequencies=[]  Unit=1  AffineConversion=off
  Product : Product
  Simulink-PS Converter : nesl_utility/Simulink-PS Converter  PhysicalDomain=network_engine_domain  SubClassName=ps_input  LeftPortType=input  RightPortType=output  PseudoPeriodic=off  Frequencies=[]  NoiseDistribution=none  NoiseParameters=[]  Unit=1  AffineConversion=off  InputFiltering=off  SimscapeFilterOrder=1  InputFilterTimeConstant=0.001  UdotUserProvided=1
  Variable Resistor : fl_lib/Electrical/Electrical Elements/Variable Resistor  Rmin=100 Ohm  i_specify=off  i_priority=High  i=0 A  v_specify=off  v_priority=High  v=0 V
  In : PMIOPort  Port=1  Side=Left
  Out : PMIOPort  Port=2  Side=Right
  wires:
  Gain/1 -> Integrator/1
  Product/1 -> Gain/1
  Integrator/1 -> Fcn1/1, Fcn/1
  Fcn/1 -> Product/2
  Fcn1/1 -> Simulink-PS Converter/1
  PS-Simulink Converter/1 -> Product/1
  connections:
  Current Sensor/RConn1 -- PS-Simulink Converter/LConn1
  Current Sensor/RConn2 -- Out/RConn1
  Variable Resistor/LConn2 -- In/RConn1
  Simulink-PS Converter/RConn1 -- Variable Resistor/LConn1
  Variable Resistor/RConn1 -- Current Sensor/LConn1
